simulink model "snn_lib_dataset_test"  (R2026a)
settings: Solver=FixedStepDiscrete  FixedStep=1
libraries: snn_champions_lib x8
settings Model: Creator=user poco smart  LastModifiedBy=user poco smart

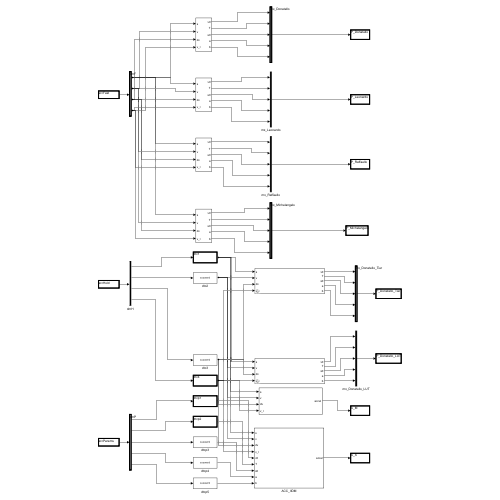
[thumbnail: Simulink's stored preview of the top-level diagram]
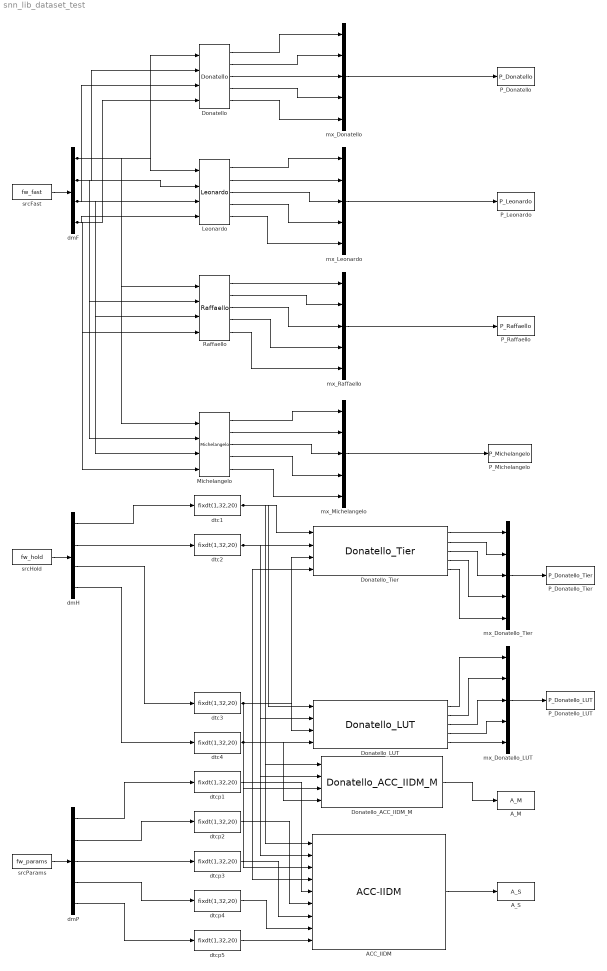
== system snn_lib_dataset_test ==
  ACC_IIDM : snn_champions_lib/ACC-IIDM  Description=|  SystemSampleTime=-1  VariantActivationTime=update diagram  EmptyChoice=off  PassThrough=off  PassThroughVariantControl=(default)  EmptyChoiceVariantControl=(default)  AllowFlexibleInterface=on  Latency=0  AutoFrameSizeCalculation=off
      | ACC-IIDM - controllore IIDM standalone (car-following), architettura R17, HDL-ready.
      | 
      | FUNZIONE: riceve i 5 parametri IDM (v0,T,s0,a,b) + lo stato (s,v,dv,v_l) e calcola l'accelerazione.
      | NON contiene la SNN -> componibile con qualunque estimator (es. Donatello_Tier). E' la chart di
      | Donatello_ACC_IIDM_M SENZA la SNN, bit-exact vs acc_iidm_open (dmax=0, run_iidm_r17_func_gate).
      | 
      | ARCHITETTURA R17 (hdl_iidm/RESULTS.txt): divisore e radice digit-recurrence SEQUENZIALI (hardware piu'
      | piccolo del combinatorio), USE/FINAL/PREP a stadi. Fmax standalone 75,6 MHz OOC reg-reg (il controllore
      | completo 77,9). nfrac=8 (precisione fissa R17); sweet spot confermato da Quantizzation_Study_IIDM.
      | 
      | INGRESSI (9, fisici, fixed >=20 bit fraz. - interporre un Data Type Conversion):
      |   s, v, dv (= v - v_l), v_l, v0, T, s0, a, b   ->   USCITA: accel [m/s^2].
      | 
      | RATE: ~150 clock/inferenza (time-mux), edge-triggered (1 cambio ingressi = 1 inferenza, l'uscita tiene).
      | Sull'FPGA irrilevante (control-step 0,1 s = 800.000 clock @8 MHz). Self-contained. Rigen.: build_acc_iidm_block.m.
      settings: SourceProductName=SNN_Library
  A_M : ToWorkspace  VariableName=A_M  SampleTime=-1
  A_S : ToWorkspace  VariableName=A_S  SampleTime=-1
  Donatello : snn_champions_lib/Donatello  Description=|  SystemSampleTime=-1  VariantActivationTime=update diagram  EmptyChoice=off  PassThrough=off  PassThroughVariantControl=(default)  EmptyChoiceVariantControl=(default)  AllowFlexibleInterface=on  Latency=0  AutoFrameSizeCalculation=off
      | Donatello - champion SNN car-following, forward ALIF in DOUBLE (riferimento comportamentale).
      | 
      | FUNZIONE: stima i 5 parametri IDM (v0, T, s0, a, b) dallo stato di car-following (s, v, dv, v_l).
      | E' il forward del champion in doppia precisione (pesi bakati + normalizzazione + ALIF 10 tick + decode),
      | self-contained. Serve da RIFERIMENTO: i blocchi HDL (Donatello_LUT/Tier, ACC-IIDM) sono la versione
      | fixed-point di questo forward.
      | 
      | SEMANTICA: 1 campione = 1 inferenza (stato ALIF persistente sulla traiettoria). NON e' HDL-ready: e'
      | la versione double comportamentale. I/O fisico: s,v,dv,v_l -> v0,T,s0,a,b. Rigenerazione: build_library.m.
      settings: SourceProductName=SNN_Library
  Donatello_ACC_IIDM_M : snn_champions_lib/Donatello_ACC_IIDM_M  Description=|  SystemSampleTime=-1  VariantActivationTime=update diagram  EmptyChoice=off  PassThrough=off  PassThroughVariantControl=(default)  EmptyChoiceVariantControl=(default)  AllowFlexibleInterface=on  Latency=0  AutoFrameSizeCalculation=off
      | Donatello_ACC_IIDM_M - Donatello (LUT-64) + ACC-IIDM, architettura R17 (controllore completo SNN+IIDM).
      | 
      | Divisore e radice (s_star) dell'IIDM = digit-recurrence SEQUENZIALI (1-2 bit/ciclo) orchestrati da una
      | FSM a stadi (1 op/fase, registro fra le fasi). Campagna hdl_iidm/RESULTS.txt: 17 round bit-exact, Fmax OOC
      | xc7z020 R0 15,7 -> R17 77,9 MHz (+397%), 8387 LUT / 4069 FF / 68 DSP, collo st_a_iidm (14 liv).
      | ATTENZIONE: 77,9 MHz e' OOC reg-reg (NON io-timed): il deployabile e' inferiore; conta il MARGINE sul
      | control-step (~358 clock su 800.000 @8 MHz), non il valore assoluto. Bit-identico a SP3 (dmax=0).
      | Self-contained + HDL-ready. Ingressi fisici fixed >=20 bit fraz.: s,v,dv,v_l -> accel.
      | Rigenerazione: build_hdl_variants.m (+ reorg_library.m per togliere i singoli).
      settings: SourceProductName=SNN_Library
  Donatello_LUT : snn_champions_lib/Donatello_LUT  NLUT=64
      settings: SourceProductName=SNN_Library
  Donatello_Tier : snn_champions_lib/Donatello_Tier  TIER=BALANCED  NFRAC=13  ADV=off  nV=13  nfat=13  nacc=13  naccw=13  nraw=13  nw=13
      settings: SourceProductName=SNN_Library
  Leonardo : snn_champions_lib/Leonardo  Description=|  SystemSampleTime=-1  VariantActivationTime=update diagram  EmptyChoice=off  PassThrough=off  PassThroughVariantControl=(default)  EmptyChoiceVariantControl=(default)  AllowFlexibleInterface=on  Latency=0  AutoFrameSizeCalculation=off
      | Leonardo - champion SNN car-following, forward ALIF in DOUBLE (riferimento comportamentale).
      | 
      | FUNZIONE: stima i 5 parametri IDM (v0, T, s0, a, b) dallo stato di car-following (s, v, dv, v_l).
      | E' il forward del champion in doppia precisione (pesi bakati + normalizzazione + ALIF 10 tick + decode),
      | self-contained. Serve da RIFERIMENTO: i blocchi HDL (Donatello_LUT/Tier, ACC-IIDM) sono la versione
      | fixed-point di questo forward.
      | 
      | SEMANTICA: 1 campione = 1 inferenza (stato ALIF persistente sulla traiettoria). NON e' HDL-ready: e'
      | la versione double comportamentale. I/O fisico: s,v,dv,v_l -> v0,T,s0,a,b. Rigenerazione: build_library.m.
      settings: SourceProductName=SNN_Library
  Michelangelo : snn_champions_lib/Michelangelo  Description=|  SystemSampleTime=-1  VariantActivationTime=update diagram  EmptyChoice=off  PassThrough=off  PassThroughVariantControl=(default)  EmptyChoiceVariantControl=(default)  AllowFlexibleInterface=on  Latency=0  AutoFrameSizeCalculation=off
      | Michelangelo - champion SNN car-following, forward ALIF in DOUBLE (riferimento comportamentale).
      | 
      | FUNZIONE: stima i 5 parametri IDM (v0, T, s0, a, b) dallo stato di car-following (s, v, dv, v_l).
      | E' il forward del champion in doppia precisione (pesi bakati + normalizzazione + ALIF 10 tick + decode),
      | self-contained. Serve da RIFERIMENTO: i blocchi HDL (Donatello_LUT/Tier, ACC-IIDM) sono la versione
      | fixed-point di questo forward.
      | 
      | SEMANTICA: 1 campione = 1 inferenza (stato ALIF persistente sulla traiettoria). NON e' HDL-ready: e'
      | la versione double comportamentale. I/O fisico: s,v,dv,v_l -> v0,T,s0,a,b. Rigenerazione: build_library.m.
      settings: SourceProductName=SNN_Library
  P_Donatello : ToWorkspace  VariableName=P_Donatello  SampleTime=-1
  P_Donatello_LUT : ToWorkspace  VariableName=P_Donatello_LUT  SampleTime=-1
  P_Donatello_Tier : ToWorkspace  VariableName=P_Donatello_Tier  SampleTime=-1
  P_Leonardo : ToWorkspace  VariableName=P_Leonardo  SampleTime=-1
  P_Michelangelo : ToWorkspace  VariableName=P_Michelangelo  SampleTime=-1
  P_Raffaello : ToWorkspace  VariableName=P_Raffaello  SampleTime=-1
  Raffaello : snn_champions_lib/Raffaello  Description=|  SystemSampleTime=-1  VariantActivationTime=update diagram  EmptyChoice=off  PassThrough=off  PassThroughVariantControl=(default)  EmptyChoiceVariantControl=(default)  AllowFlexibleInterface=on  Latency=0  AutoFrameSizeCalculation=off
      | Raffaello - champion SNN car-following, forward ALIF in DOUBLE (riferimento comportamentale).
      | 
      | FUNZIONE: stima i 5 parametri IDM (v0, T, s0, a, b) dallo stato di car-following (s, v, dv, v_l).
      | E' il forward del champion in doppia precisione (pesi bakati + normalizzazione + ALIF 10 tick + decode),
      | self-contained. Serve da RIFERIMENTO: i blocchi HDL (Donatello_LUT/Tier, ACC-IIDM) sono la versione
      | fixed-point di questo forward.
      | 
      | SEMANTICA: 1 campione = 1 inferenza (stato ALIF persistente sulla traiettoria). NON e' HDL-ready: e'
      | la versione double comportamentale. I/O fisico: s,v,dv,v_l -> v0,T,s0,a,b. Rigenerazione: build_library.m.
      settings: SourceProductName=SNN_Library
  dmF : Demux
  dmH : Demux
  dmP : Demux  Outputs=5
  dtc{1..4} (4 alike) : DataTypeConversion  OutDataTypeStr=fixdt(1,32,20)  SaturateOnIntegerOverflow=off  RndMeth=Floor
  dtcp{1..5} (5 alike) : DataTypeConversion  OutDataTypeStr=fixdt(1,32,20)  SaturateOnIntegerOverflow=off  RndMeth=Floor
  mx_Donatello : Mux  Inputs=5
  mx_Donatello_LUT : Mux  Inputs=5
  mx_Donatello_Tier : Mux  Inputs=5
  mx_Leonardo : Mux  Inputs=5
  mx_Michelangelo : Mux  Inputs=5
  mx_Raffaello : Mux  Inputs=5
  srcFast : FromWorkspace  VariableName=fw_fast  SampleTime=1  Interpolate=off  OutputAfterFinalValue=Holding final value
  srcHold : FromWorkspace  VariableName=fw_hold  SampleTime=1  Interpolate=off  OutputAfterFinalValue=Holding final value
  srcParams : FromWorkspace  VariableName=fw_params  SampleTime=1  Interpolate=off  OutputAfterFinalValue=Holding final value
  wires:
  dmF/2 -> Leonardo/2, Michelangelo/2, Raffaello/2, Donatello/2
  srcFast/1 -> dmF/1
  Raffaello/5 -> mx_Raffaello/5
  Leonardo/4 -> mx_Leonardo/4
  Donatello/5 -> mx_Donatello/5
  srcHold/1 -> dmH/1
  Leonardo/5 -> mx_Leonardo/5
  dmH/1 -> dtc1/1
  srcParams/1 -> dmP/1
  Donatello_LUT/2 -> mx_Donatello_LUT/2
  dtcp5/1 -> ACC_IIDM/9
  dmF/1 -> Leonardo/1, Donatello/1, Michelangelo/1, Raffaello/1
  mx_Michelangelo/1 -> P_Michelangelo/1
  dtcp2/1 -> ACC_IIDM/6
  dmF/3 -> Leonardo/3, Donatello/3, Raffaello/3, Michelangelo/3
  Donatello_LUT/4 -> mx_Donatello_LUT/4
  dmF/4 -> Michelangelo/4, Leonardo/4, Raffaello/4, Donatello/4
  dmH/2 -> dtc2/1
  dmH/3 -> dtc3/1
  dmH/4 -> dtc4/1
  dmP/1 -> dtcp1/1
  Raffaello/2 -> mx_Raffaello/2
  dmP/2 -> dtcp2/1
  dmP/3 -> dtcp3/1
  dtc4/1 -> Donatello_Tier/4, Donatello_LUT/4, Donatello_ACC_IIDM_M/4, ACC_IIDM/4
  dmP/4 -> dtcp4/1
  Michelangelo/4 -> mx_Michelangelo/4
  dmP/5 -> dtcp5/1
  Raffaello/1 -> mx_Raffaello/1
  Donatello/1 -> mx_Donatello/1
  Leonardo/1 -> mx_Leonardo/1
  Donatello/2 -> mx_Donatello/2
  dtc3/1 -> Donatello_LUT/3, Donatello_ACC_IIDM_M/3, ACC_IIDM/3, Donatello_Tier/3
  Raffaello/3 -> mx_Raffaello/3
  Leonardo/2 -> mx_Leonardo/2
  Donatello/3 -> mx_Donatello/3
  mx_Donatello/1 -> P_Donatello/1
  Leonardo/3 -> mx_Leonardo/3
  Donatello/4 -> mx_Donatello/4
  Raffaello/4 -> mx_Raffaello/4
  Michelangelo/1 -> mx_Michelangelo/1
  dtcp1/1 -> ACC_IIDM/5
  Michelangelo/2 -> mx_Michelangelo/2
  Michelangelo/3 -> mx_Michelangelo/3
  Michelangelo/5 -> mx_Michelangelo/5
  dtc1/1 -> Donatello_LUT/1, Donatello_Tier/1, Donatello_ACC_IIDM_M/1, ACC_IIDM/1
  dtc2/1 -> Donatello_LUT/2, Donatello_Tier/2, Donatello_ACC_IIDM_M/2, ACC_IIDM/2
  Donatello_Tier/1 -> mx_Donatello_Tier/1
  dtcp3/1 -> ACC_IIDM/7
  Donatello_Tier/5 -> mx_Donatello_Tier/5
  dtcp4/1 -> ACC_IIDM/8
  Donatello_Tier/3 -> mx_Donatello_Tier/3
  mx_Leonardo/1 -> P_Leonardo/1
  mx_Raffaello/1 -> P_Raffaello/1
  Donatello_Tier/2 -> mx_Donatello_Tier/2
  Donatello_Tier/4 -> mx_Donatello_Tier/4
  Donatello_LUT/1 -> mx_Donatello_LUT/1
  mx_Donatello_Tier/1 -> P_Donatello_Tier/1
  Donatello_LUT/3 -> mx_Donatello_LUT/3
  Donatello_LUT/5 -> mx_Donatello_LUT/5
  Donatello_ACC_IIDM_M/1 -> A_M/1
  mx_Donatello_LUT/1 -> P_Donatello_LUT/1
  ACC_IIDM/1 -> A_S/1
